simulink model "WMC_Ver_01_CoreCycle"  (R2026a)
settings: Solver=FixedStepAuto  StopTime=inf  FixedStep=0.1
settings Model: PacingRate=5  Creator=Rakshith  LastModifiedBy=Rakshith

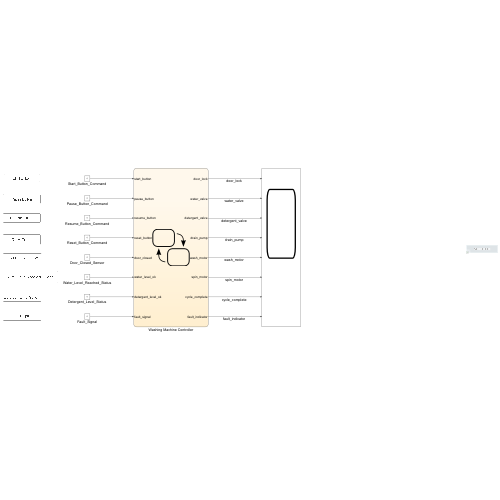
[thumbnail: Simulink's stored preview of the top-level diagram]
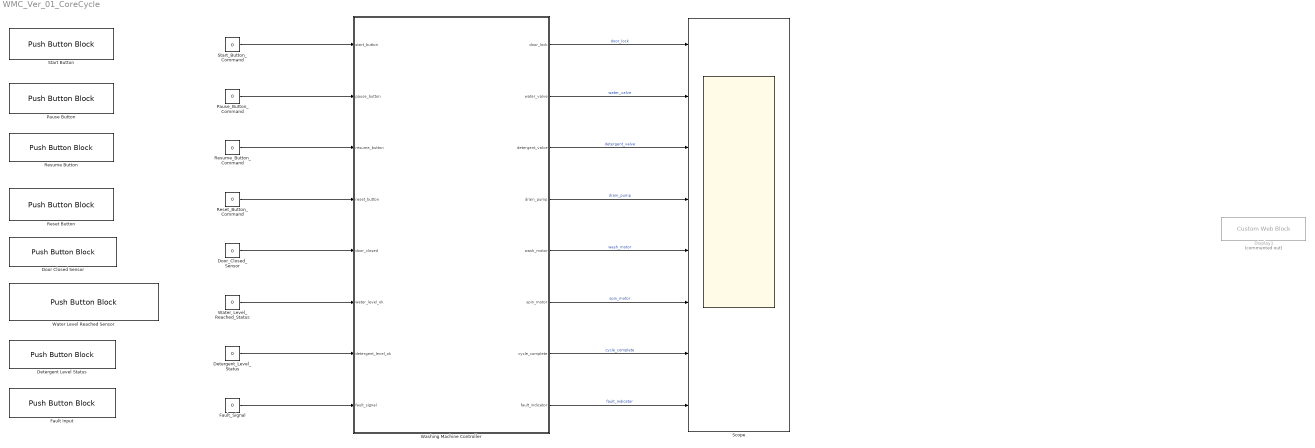
== system WMC_Ver_01_CoreCycle ==
  Detergent Level Status : PushButtonBlock  ButtonText=Detergent Level Sensor  IconOnColor=[0.0, 0.39215686274509803, 0.0]  IconOffColor=[0.0, 1.0, 0.0]  OffValue=0.000000
  Detergent_Level_Status : Constant  Value=0
  Display1 : CustomWebBlock  Commented=on  LabelPosition=Hide  ShowInitialText=on  Configuration="{\"components\":[{\"name\":\"DisplayComponent\",\"settings\":{\"alignment\":\"center\",\"bold\":false,\"font\":\"DSEG7 Classic\",\"fontColor\":[255,255,200],\"fontSize\":\"14\",\"format\":\"Custom\",\"formatString\":\"%s\",\"italic\":false,\"position\":[0,0,1,1],\"underline\":false}},{\"name\":\"BackgroundImageComponent\",\"settings\":{\"image\":{\"size\":[300,80],\"src\":\"data:image\\/svg+xml;base64,PHN2ZyBpZD0iZnJhbWUiIHhtbG5zPSJodHRwOi8vd3d3LnczLm9yZy8yMDAwL3N2ZyIgeG1sbnM6eGxpbms9Imh0dHA6Ly93d3cudzMub3JnLzE5OTkveGxpbmsiIHZpZXdCb3g9IjAgMCAzODAgMTAxIj48ZGVmcz48c3R5bGU+LmNscy0xe2ZpbGw6IzAwMmI0Mjt9LmNscy0ye2ZpbGw6IzQyNzA4Mjt9LmNscy0ze2ZpbGw6dXJsKCNyYWRpYWwtZ3JhZGllbnQpO308L3N0eWxlPjxyYWRpYWxHcmFkaWVudCBpZD0icmFkaWFsLWdyYWRpZW50IiBjeD0iMTkwIiBjeT0iNTAuNSIgcj0iMjY5LjIxIiBncmFkaWVudFVuaXRzPSJ1c2VyU3BhY2VPblVzZSI+PHN0b3Agb2Zmc2V0PSIwLjAxIiBzdG9wLWNvbG9yPSIjM2U0ZjU4Ii8+PHN0b3Agb2Zmc2V0PSIwLjA2IiBzdG9wLWNvbG9yPSIjNDQ1NzYxIi8+PHN0b3Agb2Zmc2V0PSIwLjE1IiBzdG9wLWNvbG9yPSIjNTU2YTc2Ii8+PHN0b3Agb2Zmc2V0PSIwLjI1IiBzdG9wLWNvbG9yPSIjNmQ4ODk1Ii8+PHN0b3Agb2Zmc2V0PSIwLjM4IiBzdG9wLWNvbG9yPSIjOGZiMmMzIi8+PHN0b3Agb2Zmc2V0PSIwLjUyIiBzdG9wLWNvbG9yPSIjYjZlNGZhIi8+PHN0b3Agb2Zmc2V0PSIxIiBzdG9wLWNvbG9yPSIjMTU0NjU3Ii8+PC9yYWRpYWxHcmFkaWVudD48L2RlZnM+PGcgaWQ9IkxheWVyXzIiIGRhdGEtbmFtZT0iTGF5ZXIgMiI+PGcgaWQ9IkxheWVyXzEtMiIgZGF0YS1uYW1lPSJMYXllciAxLTIiPjxyZWN0IGlkPSJyZWN0MTAzNiIgY2xhc3M9ImNscy0xIiB4PSIxMSIgeT0iMTEiIHdpZHRoPSIzNTgiIGhlaWdodD0iNzkiLz48cGF0aCBpZD0icGF0aDEwMzgiIGNsYXNzPSJjbHMtMiIgZD0iTTgsOFY5M0gzNzJWOFpNMzY5LDkwSDExVjExSDM2OVoiLz48cGF0aCBpZD0icGF0aDEwNDAiIGNsYXNzPSJjbHMtMyIgZD0iTTAsMFYxMDFIMzgwVjBaTTM3Miw5M0g4VjhIMzcyWiIvPjwvZz48L2c+PC9zdmc+\",\"srcOrientation\":\"Right\"},\"position\":[0,0,1,1],\"scaleMode\":\"0\"}},{\"name\":\"ForegroundImageComponent\",\"settings\":{\"angle\":0,\"image\":{\"size\":[0,0],\"src\":\"default\"},\"isForeground\":1,\"position\":[0,0,1,1],\"scaleMode\":\"0\"}}],\"derived\":{\"blockParameters\":{\"alignment\":\"center\",\"fixedAspectRatio\":\"on\",\"format\":\"Custom\",\"formatString\":\"%s\"}},\"settings\":{\"BindingType\":\"signal\",\"aspectRatio\":1.032258064516129,\"backgroundColor\":[0,0,0,\"1\"],\"backgroundOffset\":0.14,\"backgroundOpacity\":1,\"fixedAspectRatio\":\"on\",\"showBackgroundColor\":false,\"value\":0,\"version\":\"R2025b\"},\"type\":\"Display\"}"
  Door Closed Sensor : PushButtonBlock  ButtonText=Door Closed Sensor  IconOnColor=[0.0, 0.39215686274509803, 0.0]  IconOffColor=[0.0, 1.0, 0.0]  OffValue=0.000000
  Door_Closed_Sensor : Constant  Value=0
  Fault Input : PushButtonBlock  ButtonText=Fault Input  IconOnColor=[0.0, 0.39215686274509803, 0.0]  IconOffColor=[0.0, 1.0, 0.0]  OffValue=0.000000
  Fault_Signal : Constant  Value=0
  Pause Button : PushButtonBlock  ButtonText=Pause Button  IconOnColor=[0.0, 0.39215686274509803, 0.0]  IconOffColor=[0.0, 1.0, 0.0]  OffValue=0.000000
  Pause_Button_Command : Constant  Value=0
  Reset Button : PushButtonBlock  ButtonText=Reset Button  IconOnColor=[0.0, 0.39215686274509803, 0.0]  IconOffColor=[0.0, 1.0, 0.0]  OffValue=0.000000
  Reset_Button_Command : Constant  Value=0
  Resume Button : PushButtonBlock  ButtonText=Resume Button  IconOnColor=[0.0, 0.39215686274509803, 0.0]  IconOffColor=[0.0, 1.0, 0.0]  OffValue=0.000000
  Resume_Button_Command : Constant  Value=0
  Scope : Scope  NumInputPorts=8
      settings: ActiveDisplayYMinimum=-0.12499999999999997  ActiveDisplayYMaximum=1.125
  Start Button : PushButtonBlock  ButtonText=Start Button  ButtonType=Latch  IconOnColor=[0.0, 0.39215686274509803, 0.0]  IconOffColor=[0.0, 1.0, 0.0]  OffValue=0.000000
  Start_Button_Command : Constant  Value=0
  Washing Machine Controller : Stateflow chart  TreatAsAtomicUnit=on
  Water Level Reached Sensor : PushButtonBlock  ButtonText=Water Level Reached Sensor  IconOnColor=[0.0, 0.39215686274509803, 0.0]  IconOffColor=[0.0, 1.0, 0.0]  OffValue=0.000000
  Water_Level_Reached_Status : Constant  Value=0
  wires:
  Start_Button_Command/1 -> Washing Machine Controller/1(start_button)
  Pause_Button_Command/1 -> Washing Machine Controller/2(pause_button)
  Resume_Button_Command/1 -> Washing Machine Controller/3(resume_button)
  Reset_Button_Command/1 -> Washing Machine Controller/4(reset_button)
  Door_Closed_Sensor/1 -> Washing Machine Controller/5(door_closed)
  Water_Level_Reached_Status/1 -> Washing Machine Controller/6(water_level_ok)
  Fault_Signal/1 -> Washing Machine Controller/8(fault_signal)
  Detergent_Level_Status/1 -> Washing Machine Controller/7(detergent_level_ok)
  Washing Machine Controller/5(wash_motor) -> Scope/5  "wash_motor"
  Washing Machine Controller/1(door_lock) -> Scope/1  "door_lock"
  Washing Machine Controller/2(water_valve) -> Scope/2  "water_valve"
  Washing Machine Controller/3(detergent_valve) -> Scope/3  "detergent_valve"
  Washing Machine Controller/4(drain_pump) -> Scope/4  "drain_pump"
  Washing Machine Controller/6(spin_motor) -> Scope/6  "spin_motor"
  Washing Machine Controller/7(cycle_complete) -> Scope/7  "cycle_complete"
  Washing Machine Controller/8(fault_indicator) -> Scope/8  "fault_indicator"

== stateflow chart WMC_Ver_01_CoreCycle/Washing Machine Controller ==
  state Idle
    en: door_lock = 0;
    water_valve = 0;
    detergent_valve = 0;
    drain_pump = 0;
    wash_motor = 0;
    spin_motor = 0;
    cycle_complete = 0;
    fault_indicator = 0;
  state Door_Lock_Activation
    en: door_lock = 1;
    water_valve = 0;
    detergent_valve = 0;
    drain_pump = 0;
    wash_motor = 0;
    spin_motor = 0;
    cycle_complete = 0;
  state Water_Fill_Wash_Cycle
    en: door_lock = 1;
    water_valve = 1;
    detergent_valve = 0;
    drain_pump = 0;
    wash_motor = 0;
    spin_motor = 0;
    cycle_complete = 0;
  state Detergent_Fill
    en: door_lock = 1;
    water_valve = 0;
    detergent_valve = 1;
    drain_pump = 0;
    wash_motor = 0;
    spin_motor = 0;
    cycle_complete = 0;
  state Wash
    en: door_lock = 1;
    water_valve = 0;
    detergent_valve = 0;
    drain_pump = 0;
    wash_motor = 1;
    spin_motor = 0;
    cycle_complete = 0;
  state Drain_Wash_Cycle
    en: door_lock = 1;
    water_valve = 0;
    detergent_valve = 0;
    drain_pump = 1;
    wash_motor = 0;
    spin_motor = 0;
    cycle_complete = 0;
  state Water_Fill_Rinse_Cycle
    en: door_lock = 1;
    water_valve = 1;
    detergent_valve = 0;
    drain_pump = 0;
    wash_motor = 0;
    spin_motor = 0;
    cycle_complete = 0;
  state Rinse
    en: door_lock = 1;
    water_valve = 0;
    detergent_valve = 0;
    drain_pump = 0;
    wash_motor = 1;
    spin_motor = 0;
    cycle_complete = 0;
  state Cycle_Complete
    en: door_lock = 0;
    water_valve = 0;
    detergent_valve = 0;
    drain_pump = 0;
    wash_motor = 0;
    spin_motor = 0;
    cycle_complete = 1;
  state Drain_Rinse_Cycle
    en: door_lock = 1;
    water_valve = 0;
    detergent_valve = 0;
    drain_pump = 1;
    wash_motor = 0;
    spin_motor = 0;
    cycle_complete = 0;
  state Spin
    en: door_lock = 1;
    water_valve = 0;
    detergent_valve = 0;
    drain_pump = 0;
    wash_motor = 0;
    spin_motor = 1;
    cycle_complete = 0;
  (default) -> Idle
  Cycle_Complete -> Idle : [after(10, sec)]
  Door_Lock_Activation -> Idle [order 1] : [door_closed == 0]
  Idle -> Door_Lock_Activation : [start_button == 1 && door_closed == 1]
  Water_Fill_Wash_Cycle -> Detergent_Fill : [water_level_ok == 1]
  Detergent_Fill -> Wash : [detergent_level_ok == 1]
  Door_Lock_Activation -> Water_Fill_Wash_Cycle [order 2] : [after(door_lock_delay, sec) && door_closed ==1]
  Wash -> Drain_Wash_Cycle : [after(wash_duration, sec)]
  Drain_Wash_Cycle -> Water_Fill_Rinse_Cycle : [after(drain_duration, sec)]
  Water_Fill_Rinse_Cycle -> Rinse : [water_level_ok == 1]
  Rinse -> Drain_Rinse_Cycle : [after(rinse_duration, sec)]
  Drain_Rinse_Cycle -> Spin : [after(drain_duration, sec)]
  Spin -> Cycle_Complete : [after(spin_duration, sec)]
  data: door_lock output; water_valve output; start_button input; pause_button input; resume_button input; reset_button input; door_closed input; water_level_ok input; detergent_level_ok input; detergent_valve output; drain_pump output; wash_motor output; spin_motor output; cycle_complete output; fault_indicator output; wash_duration local =20*60; drain_duration local =4*60; rinse_duration local =15*60; spin_duration local =10*60; door_lock_delay local =10; fault_signal input; detergent_fill_timeout local
